simulink model "ex3_a"  (R2023b)
settings: Solver=VariableStepAuto  StartTime=0.0  StopTime=500  RelTol=1e-3
values from neighbouring files (symbols this model uses):
  kI = 2    [tema7_ts.m]
  kP = 2    [tema7_ts.m]
  kR = 8    [tema7_ts.m]
settings Model: Creator=chapo  LastModifiedBy=chapo

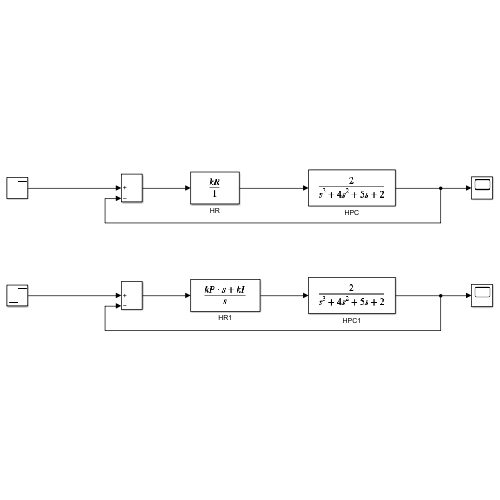
[thumbnail: Simulink's stored preview of the top-level diagram]
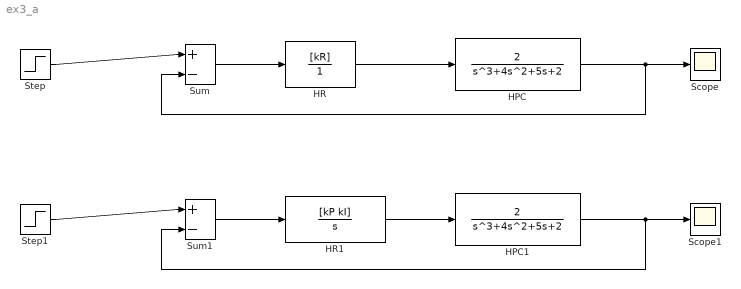
== system ex3_a ==
  HPC : TransferFcn  Numerator=[2]  Denominator=[1 4 5 2]
  HPC1 : TransferFcn  Numerator=[2]  Denominator=[1 4 5 2]
  HR : TransferFcn  Numerator=[kR]  Denominator=1
  HR1 : TransferFcn  Numerator=[kP kI]  Denominator=[1 0]
  Scope : Scope
  Scope1 : Scope
  Step : Step  SampleTime=0
  Step1 : Step  SampleTime=0
  Sum : Sum  Inputs=|+-
  Sum1 : Sum  Inputs=|+-
  wires:
  Sum/1 -> HR/1
  Step/1 -> Sum/1
  HR/1 -> HPC/1
  HPC/1 -> Sum/2, Scope/1
  HPC1/1 -> Sum1/2, Scope1/1
  HR1/1 -> HPC1/1
  Step1/1 -> Sum1/1
  Sum1/1 -> HR1/1
